simulink model "sih_planner"  (R2026a)
settings: Solver=FixedStepDiscrete  FixedStep=0.01
settings Model: Creator=user  LastModifiedBy=user

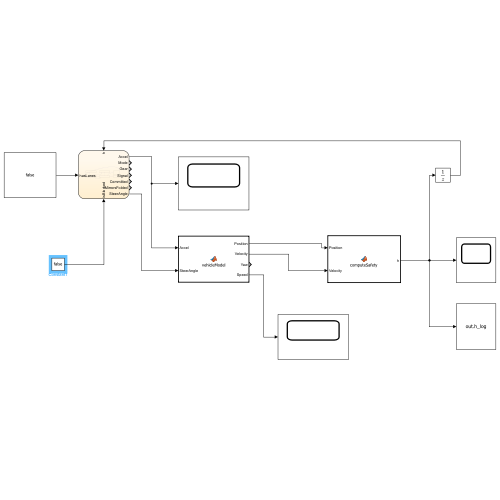
[thumbnail: Simulink's stored preview of the top-level diagram]
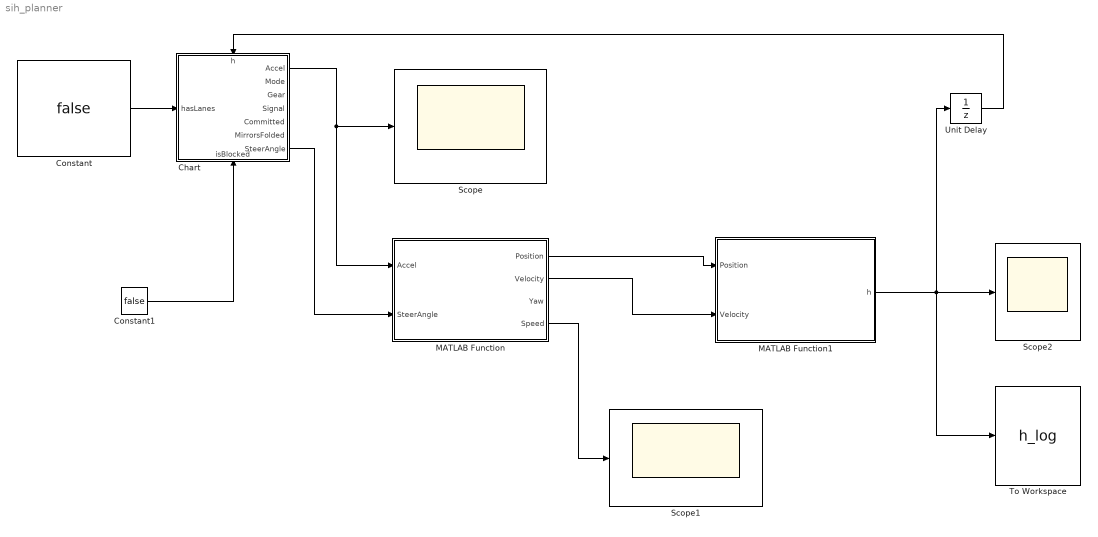
== system sih_planner ==
  Chart : Stateflow chart  TreatAsAtomicUnit=on
      settings: PortSchema="{\"entries\":[{\"content\":{\"sides\":[{\"content\":{\"connectorIds\":[\"In1\"]},\"type\":\"ConnectorPlacement.EquallySpacedRectSide\",\"uuid\":\"54091adf-f7b5-449a-85a0-6732c35b5556\"},{\"content\":{\"connectorIds\":[\"Out1\",\"Out2\",\"Out3\",\"Out5\",\"Out6\",\"Out7\",\"Out4\"],\"side\":\"RIGHT\"},\"type\":\"ConnectorPlacement.EquallySpacedRectSide\",\"uuid\":\"7677b010-2ee2-4be5-bf68-8403b0fca5c4\"},{\"content\":{\"connectorIds\":[\"In2\"],\"side\":\"TOP\"},\"type\":\"ConnectorPlacement.EquallySpacedRectSide\",\"uuid\":\"f4f99cd9-354e-4fbd-bae0-c0029e96153c\"},{\"content\":{\"connectorIds\":[\"In3\"],\"side\":\"BOTTOM\"},\"type\":\"ConnectorPlacement.EquallySpacedRectSide\",\"uuid\":\"042ef080-1598-42e3-831d-3b0f97ac8d93\"}]},\"type\":\"ConnectorPlacement.EquallySpacedConnector\",\"uuid\":\"443e1c87-78e7-485c-8e89-aa3bee582faa\"}],\"packageUris\":[\"http://schema.mathworks.com/mf0/Connector/R2020b\"],\"version\":\"1.0\"}"
  Constant : Constant  Value=false  OutDataTypeStr=boolean
  Constant1 : Constant  Value=false
  MATLAB Function : MATLAB Function  TreatAsAtomicUnit=on
  MATLAB Function1 : MATLAB Function  TreatAsAtomicUnit=on
  Scope : Scope
      settings: ActiveDisplayYMinimum=-1  ActiveDisplayYMaximum=1
  Scope1 : Scope
      settings: ActiveDisplayYMinimum=-0.86144240560351593  ActiveDisplayYMaximum=6.1128823322571639
  Scope2 : Scope
      settings: ActiveDisplayYMinimum=0.029930897398311125  ActiveDisplayYMaximum=0.049930897398311129  DataLoggingVariableName=ScopeData2
  To Workspace : ToWorkspace  VariableName=h_log  SaveFormat=Timeseries  SampleTime=-1
  Unit Delay : UnitDelay  InitialCondition=1.0  SampleTime=-1
  wires:
  Chart/1(Accel) -> MATLAB Function/1(Accel), Scope/1
  Chart/4(SteerAngle) -> MATLAB Function/2(SteerAngle)
  MATLAB Function/4(Speed) -> Scope1/1
  MATLAB Function/1(Position) -> MATLAB Function1/1(Position)
  MATLAB Function/2(Velocity) -> MATLAB Function1/2(Velocity)
  MATLAB Function1/1(h) -> To Workspace/1, Unit Delay/1, Scope2/1
  Constant/1 -> Chart/1(hasLanes)
  Unit Delay/1 -> Chart/2(h)
  Constant1/1 -> Chart/3(isBlocked)

== matlab function sih_planner/MATLAB Function1 ==
  data: Position input; h output; Velocity input
function h = computeSafety(Position, Velocity)
%#codegen
% Computes h = lambda - beta for one fake agent.
% Matches the tested formulation in velocityObstacle.m.
% h >= 0 means safe. h < 0 means collision course.

    % --- FAKE TRACK LIST (stub for Aditya's perception) ---
    % One car ahead at x=50, moving toward us at 5 m/s.
    agentPos = [50, 5, 0];      % metres, ego frame
    agentVel = [-5, 0, 0];      % m/s, coming toward us

    dMin = 3.0;                  % minimum safe distance, metres

    % --- Relative geometry ---
    r  = agentPos(1:2) - Position(1:2);    % relative position (2D)
    vr = Velocity(1:2) - agentVel(1:2);    % relative velocity (2D)
    d  = sqrt(r(1)^2 + r(2)^2);           % distance

    % If within dMin, we are colliding: h = -pi/2 (do not compute lambda)
    if d <= dMin
        h = -pi/2;
        return;
    end

    % beta: half-angle of the danger cone
    beta = asin(min(dMin / d, 1.0));

    % lambda: angle between relative velocity and line of sight
    vr_mag = sqrt(vr(1)^2 + vr(2)^2);
    if vr_mag < 0.001
        h = pi - beta;   % no relative motion, very safe
        return;
    end

    cosLambda = (vr(1)*r(1) + vr(2)*r(2)) / (vr_mag * d);
    cosLambda = max(min(cosLambda, 1.0), -1.0);
    lambda = acos(cosLambda);

    h = lambda - beta;
end

== matlab function sih_planner/MATLAB Function ==
  data: Accel input; Position output; SteerAngle input; Velocity output; Yaw output; Speed output
function [Position, Velocity, Yaw, Speed] = vehicleModel(Accel, SteerAngle)
%#codegen
% Simple bicycle kinematic model.
% Uses persistent variables to remember state between time steps.

    L = 2.7;          % wheelbase in metres (typical car)
    dt = 0.01;        % time step in seconds

    persistent x y yaw speed
    if isempty(x)
        x = 0; y = 0; yaw = 0; speed = 0;
    end

    % Update speed (clamp to >= 0, car does not reverse yet)
    speed = speed + Accel * dt;
    speed = max(speed, 0);

    % Update yaw (heading direction)
    if speed > 0.01
        yaw = yaw + (speed * tan(SteerAngle) / L) * dt;
    end

    % Update position
    x = x + speed * cos(yaw) * dt;
    y = y + speed * sin(yaw) * dt;

    % Pack outputs matching egoState shape from AGENTS.md S4
    Position = [x, y, 0];
    Velocity = [speed * cos(yaw), speed * sin(yaw), 0];
    Yaw = yaw;
    Speed = speed;
end

== stateflow chart sih_planner/Chart ==
  state STRUCTURED
    entry: Accel = 0; SteerAngle = 0; Mode = uint8(0); Gear = int8(1);
    entry: Signal = uint8(0); Committed = false; MirrorsFolded = false;
  state HANDOVER
    entry: Accel = 0; SteerAngle = 0; Mode = uint8(1); Gear = int8(0);
    entry: Signal = uint8(6); Committed = false; MirrorsFolded = false;
  state EMERGENCY
    entry:
    Accel = -6.0;
    SteerAngle = 0;
    Mode = uint8(2);
    Gear = int8(0);
    Signal = uint8(3);
    Committed = false;
    MirrorsFolded = false;
  state IDLE
    entry: Accel = 0; SteerAngle = 0; Mode = uint8(1); Gear = int8(0);
    entry: Signal = uint8(0); Committed = false; MirrorsFolded = false;
  state CREEP
    entry: Accel = 0.5; SteerAngle = 0; Mode = uint8(1); Gear = int8(1);
    entry: Signal = uint8(0); Committed = false; MirrorsFolded = false;
  state COMMIT
    entry: Accel = 1.5; SteerAngle = 0; Mode = uint8(1); Gear = int8(1);
    entry: Signal = uint8(0); Committed = true; MirrorsFolded = false;
  state DONE
    entry: Accel = 0; SteerAngle = 0; Mode = uint8(1); Gear = int8(0);
    entry: Signal = uint8(0); Committed = false; MirrorsFolded = false;
  EMERGENCY -> IDLE : [h > 0.5]
  CREEP -> EMERGENCY [order 4] : [h < 0]
  IDLE -> STRUCTURED [order 2] : [hasLanes]
  IDLE -> HANDOVER [order 3] : [isBlocked && ~Committed]
  CREEP -> HANDOVER [order 3] : [isBlocked && ~Committed]
  (default) -> IDLE
  COMMIT -> EMERGENCY [order 2] : [h < 0]
  CREEP -> COMMIT [order 1] : [after(3, sec)]
  IDLE -> CREEP [order 1] : [after(1, sec)]
  COMMIT -> DONE [order 1] : [after(2, sec)]
  CREEP -> IDLE [order 2] : [after(5, sec)]
  data: Accel output; Mode output; Gear output; SteerAngle output; Signal output; Committed output; MirrorsFolded output; hasLanes input boolean; h input double; isBlocked input boolean
